simulink model "vertical_smm_3d_with_xz_lqr_with_torque_cmds"  (R2015a)
settings: Solver=FixedStepDiscrete  SolverMode=SingleTasking  StartTime=0.0  StopTime=inf  FixedStep=sample_time  RelTol=1e-3
values from neighbouring files (symbols this model uses):
  forward_dx_of_dxstar = [-1.33147741515 -1.28147741462 -1.23147741409 -1.18147741356 -1.13147741303 -1.0814774125 -1.03147741197 -0.981477411445 -0.931477410916 -0.881477410388 -0.831477409975 -0.781477409737 ... (28413 elements, 41x21x33)]    [ref_trajs.mat]
  forward_x_of_dxstar = [0.245075236011 0.237749717983 0.230424199955 0.223098681927 0.215773163898 0.20844764587 0.201122127842 0.193796609813 0.186471091785 0.179145573757 0.171820055745 0.164494537786 ... (28413 elements, 41x21x33)]    [ref_trajs.mat]
  target_dx_range = [-1 -0.95 -0.9 -0.85 -0.8 -0.75 -0.7 -0.65 -0.6 -0.55 -0.5 -0.45 ... (41 elements, 1x41)]    [ref_trajs.mat]
undefined symbols (not defined in the file or in its folder): A_kalman_fourbar_gear, A_kalman_transverse, A_kalman_vertical, A_lpf_accelerometer, A_lpf_dtau, A_lpf_fourbar_angles, A_lpf_imu, A_lpf_lateral_angle, A_lpf_leg_spring, B1_lpf_accelerometer, B1_lpf_dtau, B1_lpf_fourbar_angles, B1_lpf_imu, B1_lpf_lateral_angle, B1_lpf_leg_spring, B2_lpf_accelerometer, B2_lpf_dtau, B2_lpf_fourbar_angles, B2_lpf_imu, B2_lpf_lateral_angle, B2_lpf_leg_spring, B_dx_versus_x0, B_kalman_fourbar_gear, B_kalman_transverse, B_kalman_vertical, backwards_K_sag_of_t, backwards_P_sag_of_t, C_kalman_fourbar_gear, C_kalman_transverse, C_kalman_vertical, com_leg_motor, com_torso, contact_threshold, control_start_time, d_ankle_to_foot, d_vertical_com, desired_com_forward_velocity, desired_com_lateral_velocity, desired_initial_leg_roll_left, desired_initial_leg_roll_right, desired_stance_beta2, desired_standing_torso_pitch, desired_standing_torso_roll, desired_standing_z, desired_torso_pitch, desired_torso_roll, Discrete, enable_bouncing, enable_hopping, fcut_contact, g, HIP_MTR_MAX_CONT_TORQUE, HIP_MTR_MAX_TORQUE, i_leg_motor, i_robot, i_torso, initial_dx_estimate, initial_dy_estimate, initial_dz_estimate, initial_leg_selection ... (+77)
libraries: simulink x18, ctrlSharedLib x7
(part 5 of 5)

== matlab function vertical_smm_3d_with_xz_lqr_with_torque_cmds/Control/Behavior Control/Primary and Lateral Behavior/Stance/3D Inverse Dynamics yawed ==
  data: right_or_left input; primary_leg_torque output double size=1; torso_roll input double size=2; torso_pitch input double size=2; torso_yaw input size=2; primary_sagittal_leg_angle input size=2; primary_leg_length input size=2; primary_leg_roll input size=2; secondary_leg_roll input size=2; GRF_desired input double size=3; ddRoll_desired input double size=1; g parameter; primary_lateral_torque output double size=1; secondary_lateral_torque output double size=1; primary_leg_force output double size=1; m_leg_motor parameter; m_torso parameter; i_torso parameter; i_leg_motor parameter; lateral_offset parameter; com_torso parameter; torso_centerline_roll_offset_angle parameter
%% Inverse dynamics
function [primary_leg_torque, primary_lateral_torque, secondary_lateral_torque, primary_leg_force]  =  InverseDynamics3D(right_or_left,...
                                                                                                                         torso_roll, torso_pitch, torso_yaw, ...
                                                                                                                         primary_sagittal_leg_angle, primary_leg_length, ...
                                                                                                                         primary_leg_roll, secondary_leg_roll, ...
                                                                                                                         GRF_desired, ddRoll_desired, ...
                                                                                                                         g, m_leg_motor, m_torso, i_torso, i_leg_motor, lateral_offset, com_torso, torso_centerline_roll_offset_angle)

    d = norm(com_torso(2:3));
    It = mean(i_torso);
    Im = mean(i_leg_motor);
    
    phi    = torso_roll(1) + torso_centerline_roll_offset_angle; % roll
    theta  = torso_pitch(1);                   % pitch
    alpha1 = primary_sagittal_leg_angle(1);    % primary sagittal leg angle
    beta1  = primary_leg_roll(1);              % primary leg roll
    beta2  = secondary_leg_roll(1);            % secondary leg roll
    if right_or_left
        beta1 = beta1 - torso_centerline_roll_offset_angle;
        beta2 = beta2 + torso_centerline_roll_offset_angle;
    else
        beta1 = beta1 + torso_centerline_roll_offset_angle;
        beta2 = beta2 - torso_centerline_roll_offset_angle;
    end 
    l1     = primary_leg_length(1);            % primary leg length
    
    dphi    = torso_roll(2);
    dtheta  = torso_pitch(2);
    dpsi    = torso_yaw(2);
    dalpha1 = primary_sagittal_leg_angle(2);
    dbeta1  = primary_leg_roll(2);
    dbeta2  = secondary_leg_roll(2);
    dl1     = primary_leg_length(2);

    Fx = GRF_desired(1);
    Fy = GRF_desired(2);
    Fz = GRF_desired(3);
    ddphi = ddRoll_desired;

    if right_or_left == 1
      A = A_id_roll_yawed_right(lateral_offset,d,m_leg_motor,m_torso,It,Im,phi,theta,alpha1,beta1,beta2,l1);     
      B = B_id_roll_yawed_right(lateral_offset,d,g,m_leg_motor,m_torso,It,Im,phi,theta,alpha1,beta1,beta2,l1,dphi,dtheta,dpsi,dalpha1,dbeta1,dbeta2,dl1,Fx,Fy,Fz,ddphi);
    else
      A = A_id_roll_yawed_left(lateral_offset,d,m_leg_motor,m_torso,It,Im,phi,theta,alpha1,beta1,beta2,l1);     
      B = B_id_roll_yawed_left(lateral_offset,d,g,m_leg_motor,m_torso,It,Im,phi,theta,alpha1,beta1,beta2,l1,dphi,dtheta,dpsi,dalpha1,dbeta1,dbeta2,dl1,Fx,Fy,Fz,ddphi);
    end        
    
    x_id_roll = A \ B;
    primary_leg_torque = x_id_roll(10);
    primary_lateral_torque = x_id_roll(11);
    secondary_lateral_torque = x_id_roll(12);
    primary_leg_force = x_id_roll(13);
end

== matlab function vertical_smm_3d_with_xz_lqr_with_torque_cmds/Control/Behavior Control/Primary and Lateral Behavior/Stance/COM X,Y,Z  trajectory generation ==
  data: stance input; hopping input; bouncing input; x_0 output size=1; y_0 output size=1; z_ref output size=1; dz_ref output size=1; ddz_ref output size=1; x_ref output size=1; dx_ref output size=1; y_ref output size=1; dy_ref output size=1; t input size=1; dx0 input; dy0 input; target_DX input; target_DY input; z_rest_new parameter; z_amplitude parameter; spring_frequency parameter; phase_0 parameter; forward_x_of_dxstar parameter; forward_dx_of_dxstar parameter; target_dx_range parameter; T_s parameter; desired_standing_z parameter; standing_bounce_amplitude parameter; standing_bounce_w input; standing_bounce_dw input
%% COM trajectory generation for stance & foot placement for flight

% Outputs:
% x_0: desired x position for COM at touchdown
% y_0: desired y position for COM at touchdown
% [z_ref, dz_ref, ddz_ref]: reference trajectory for vertical
% [x_ref, dx_ref]: reference trajectory for forward
% [y_ref, dy_ref]: reference trajectory for lateral

% Inputs:
% t: time since touchdown
% dx0: touchdown x velocity
% dy0: touchdown y velocity
% target_DX: desired x velocity at takeoff
% s_duration: nominal stance time
% z_rest_new: z height of oscillation
% target_dx_range: full range of possible x velocities in lookup table
% forward_x_of_dxstar: master lookup table for x trajectories
% T_s: tabled vector from 0 to s_duration

function [x_0, y_0,...
          z_ref, dz_ref, ddz_ref, ...
          x_ref, dx_ref, y_ref, dy_ref] ...
          = ReferenceTrajectory(stance, hopping, bouncing, t, dx0, dy0, target_DX, target_DY, z_rest_new, z_amplitude, ...
            spring_frequency, phase_0, forward_x_of_dxstar, forward_dx_of_dxstar, ...
            target_dx_range, T_s,...
            desired_standing_z, standing_bounce_amplitude, standing_bounce_w, standing_bounce_dw)
    
    % Z trajectory 
    z_ref =  z_rest_new + z_amplitude*sin(spring_frequency*t+phase_0);
    dz_ref = z_amplitude*spring_frequency*cos(spring_frequency*t+phase_0);
    ddz_ref = -z_amplitude*spring_frequency^2*sin(spring_frequency*t+phase_0);
    
    % saturate t and initial velocity to reference library
    t_sat = max( min(t, T_s(end)), 0);

    % [X, dX] trajectory from 0 to s_duration
    forward_x_given_dxstar = squeeze(interp1(target_dx_range, forward_x_of_dxstar, target_DX));
    forward_dx_given_dxstar = squeeze(interp1(target_dx_range, forward_dx_of_dxstar, target_DX));

    dx0 = max( min(dx0, max(forward_dx_given_dxstar(:,1))), min(forward_dx_given_dxstar(:,1)) );
    x_ref  = interp2(T_s, forward_dx_given_dxstar(:,1), forward_x_given_dxstar, t_sat, dx0);
    dx_ref = interp2(T_s, forward_dx_given_dxstar(:,1), forward_dx_given_dxstar, t_sat, dx0);
    x_0 = interp1(forward_dx_given_dxstar(:,1), forward_x_given_dxstar(:,1), dx0);

    % [Y, dY] trajectory from 0 to s_duration
    % Y uses same library as X
    forward_y_given_dxstar = squeeze(interp1(target_dx_range, forward_x_of_dxstar, target_DY));
    forward_dy_given_dxstar = squeeze(interp1(target_dx_range, forward_dx_of_dxstar, target_DY));

    dy0 = max( min(dy0, max(forward_dy_given_dxstar(:,1))), min(forward_dy_given_dxstar(:,1)) );
    y_ref  = interp2(T_s, forward_dy_given_dxstar(:,1), forward_y_given_dxstar, t_sat, dy0);
    dy_ref = interp2(T_s, forward_dy_given_dxstar(:,1), forward_dy_given_dxstar, t_sat, dy0);
    y_0 = interp1(forward_dy_given_dxstar(:,1), forward_y_given_dxstar(:,1), dy0);
    
    if ~hopping && ~bouncing % Standing still
        z_ref = desired_standing_z;
        dz_ref = 0;
        ddz_ref = 0;
        x_ref = 0;
        dx_ref = 0;
        y_ref = 0;
        dy_ref =0;
    elseif ~hopping && bouncing % Bouncing while standing
        z_ref = z_rest_new + standing_bounce_amplitude*sin(t*standing_bounce_w);
        dz_ref = standing_bounce_amplitude*cos(t*standing_bounce_w)*(t*standing_bounce_dw + standing_bounce_w);
        ddz_ref = standing_bounce_amplitude*(2*standing_bounce_dw*cos(t*standing_bounce_w) - (t*standing_bounce_dw + standing_bounce_w)^2*sin(t*standing_bounce_w));
        x_ref = 0;
        dx_ref = 0;
        y_ref = 0;
        dy_ref =0;
    elseif ~stance % Flight
        z_ref = 0;
        dz_ref = 0;
        ddz_ref = 0;
        x_ref = 0;
        dx_ref = 0;
        y_ref = 0;
        dy_ref =0;    
    end
  
end

== matlab function vertical_smm_3d_with_xz_lqr_with_torque_cmds/Control/Behavior Control/Primary and Lateral Behavior/Stance/Feedback for Lateral Stabilization ==
  data: feedforward_Fy output; hopping input; stance input; right_left input; rolldroll input; primary_lateral_torque_desired output; symdsym input; beta1dbeta1 input; beta2dbeta2 input; ydy_ref input; zdzddz_ref input; GRF_measured input; secondary_lateral_torque_desired output double size=1; m_torso parameter; m_leg_motor parameter; m_leg parameter; lateral_offset parameter; com_torso parameter; i_torso parameter; i_leg_motor parameter; desired_standing_torso_roll parameter; desired_torso_roll parameter; desired_stance_beta2 parameter; angular_momentum output; k_stance_torso_roll parameter; k_stance_secondary_roll parameter; g parameter; m_total_real parameter
%  x_front = [y, roll, sym, dy, droll, L]; 
function [feedforward_Fy, primary_lateral_torque_desired, secondary_lateral_torque_desired, angular_momentum]  =  ...
    FrontalStabilization(hopping, stance, right_left, rolldroll, symdsym, beta1dbeta1, beta2dbeta2, ydy_ref, zdzddz_ref, GRF_measured,...
           m_torso, m_leg_motor, m_leg, lateral_offset, com_torso, i_torso, i_leg_motor, ...
           desired_standing_torso_roll, desired_torso_roll, desired_stance_beta2, k_stance_torso_roll, k_stance_secondary_roll, g, m_total_real)
    
    % Angular momentum about the pelvis in the frontal plane
    d = norm(com_torso(2:3));
    It_f = i_torso(1);
    Im_f = i_leg_motor(1);
    angular_momentum = rolldroll(2)*(m_torso*d^2 + It_f + 2*(m_leg_motor*lateral_offset^2+ Im_f)) -symdsym(2)*(m_leg_motor*lateral_offset^2+Im_f);
    
    % Feedforward GRFy for inverse dynamics
    Fz_ref = (zdzddz_ref(3)+g)*m_total_real;
    feedforward_Fy = Fz_ref*ydy_ref(1)/zdzddz_ref(1);
    feedforward_Fy = min(max(feedforward_Fy, -0.5*abs(GRF_measured(3))), 0.5*abs(GRF_measured(3)));
    
    % Desired states
    if hopping
        desired_torso_roll_state = [desired_torso_roll; 0]; 
    else
        desired_torso_roll_state = [desired_standing_torso_roll; 0];
    end
    desired_beta2_state = [desired_stance_beta2; 0];
    
    % Motor torque commands
    ddz = GRF_measured(3) / m_total_real - g;
    gravity_comp = (m_leg_motor+m_leg)*lateral_offset*ddz;
    contact_factor = max(min(GRF_measured(3)/(m_total_real*g),1.0),0);
    secondary_lateral_torque_desired = k_stance_secondary_roll*(desired_beta2_state - beta2dbeta2);
    primary_lateral_feedback = contact_factor*k_stance_torso_roll*(desired_torso_roll_state - rolldroll);
    if right_left % Right leg beta direction is opposite torso roll
        primary_lateral_feedback = -primary_lateral_feedback;
    end
    primary_lateral_torque_desired =  primary_lateral_feedback + secondary_lateral_torque_desired;
      
    if ~stance
        primary_lateral_torque_desired = 0;
        secondary_lateral_torque_desired = 0;
        feedforward_Fy = 0;
    end
end

== matlab function vertical_smm_3d_with_xz_lqr_with_torque_cmds/Control/Behavior Control/Primary and Lateral Behavior/Stance/LQR Feedback for Desired Forward GRF ==
  data: hopping input; stance input; GRFx_desired output; netural_pitch_ff output; true_ff output; GRFx_lqr output; ddtheta_star output; ddtheta_star_neutral output; xdx input; thetadtheta input; zdz input; Fz input; xdx_ref input size=2; theta_star input; K_sag input; P_sag input; measured_GRF input; Fx_disturbance input; i_robot parameter; cost_to_go output double size=1; ang_mom output; desired_standing_torso_pitch parameter; k_LQR_sagittal_infinite parameter; P_LQR_sagittal_infinite parameter
%% LQR for x state

% stance: 1 if in stance, 0 otherwise
% xdx: [ x from stance leg to COM, dx of COM]
% thetadtheta: [pitch, dpitch]
% zdz: [z of COM, dz of COM]
% Fz: Desired z GRF
% xdx_ref: [x, dx] current reference point for COM
% theta_star: desired torso pitch
% K_sag: time dependent LQR gain


% sagittal_state: [x, pitch, dx, dptich]
% theta_star: desired torso pitch


function [GRFx_desired, netural_pitch_ff, true_ff, GRFx_lqr, ddtheta_star, ddtheta_star_neutral, cost_to_go, ang_mom]  =  ...
    LQR_Sagittal(hopping, stance, xdx, thetadtheta, zdz, Fz, xdx_ref, theta_star, K_sag, P_sag, measured_GRF, Fx_disturbance, i_robot,...
    desired_standing_torso_pitch, k_LQR_sagittal_infinite, P_LQR_sagittal_infinite)


    sagittal_state = [xdx(1); thetadtheta(1); xdx(2); thetadtheta(2)];
    netural_pitch_ff = Fz*xdx(1)/zdz(1);
    true_ff = Fz*xdx_ref(1)/zdz(1);
    
    if hopping
        sagittal_reference = [xdx_ref(1), theta_star, xdx_ref(2), 0]';
        sagittal_error = (sagittal_state - sagittal_reference);
        cost_to_go = 0.5*sagittal_error'*P_sag*sagittal_error;
        GRFx_lqr = - K_sag*sagittal_error;
        GRFx_desired = true_ff + GRFx_lqr;
    else
        sagittal_reference = [xdx_ref(1), desired_standing_torso_pitch, xdx_ref(2), 0]';
        sagittal_error = (sagittal_state - sagittal_reference);
        cost_to_go = 0.5*sagittal_error'*P_LQR_sagittal_infinite*sagittal_error;
        %GRFx_desired = i_robot/zdz(1)*(150*(thetadtheta(1)-desired_standing_torso_pitch) + 30*thetadtheta(2)) + netural_pitch_ff;
        GRFx_lqr = - k_LQR_sagittal_infinite*sagittal_error;
        GRFx_desired = GRFx_lqr;
    end
    
    GRFx_desired = GRFx_desired - Fx_disturbance;
    GRFx_desired = min(max(GRFx_desired, -0.5*abs(measured_GRF(3))), 0.5*abs(measured_GRF(3))); % saturate to friction cone
    
    if stance == 0
      GRFx_lqr = 0;
      cost_to_go = 0;
      netural_pitch_ff = 0;
      true_ff = 0;
    end
    
    % quantities for logging
    ddtheta_star_neutral = -(GRFx_lqr)*zdz(1)/i_robot;
    ddtheta_star = -(GRFx_desired - netural_pitch_ff)*zdz(1)/i_robot;
    ang_mom = i_robot*thetadtheta(2);
end

== matlab function vertical_smm_3d_with_xz_lqr_with_torque_cmds/Control/Behavior Control/Primary and Lateral Behavior/Stance/LQR Feedback for Desired Vertical GRF ==
  data: hopping input; stance input; zdzddz_ref input size=3; GRFz_desired output; GRFz_feedforward output; z_state input; leg_length input; Fz_disturbance input; k_LQR_vertical parameter; P_LQR_vertical parameter; k_vertical_winch parameter; m_total_real parameter; g parameter; cost_to_go output double size=1; max_leg_length parameter
%% LQR for z during stance

% stance: 1 if in stance, 0 otherwise
% z_state: [z, dz] current estimate
% zdzddz_ref: reference trajectory for z position, velocity, and acceleration


% GRFz_desired: desired z GRF
% cost_to_go: remaining LQR cost

function [GRFz_desired, GRFz_feedforward, cost_to_go]   =  ...
               LQR_Vertical_Height(hopping, stance, zdzddz_ref, z_state, leg_length, Fz_disturbance,...
                                   k_LQR_vertical, P_LQR_vertical, k_vertical_winch, m_total_real, g, max_leg_length)

    z_ref = zdzddz_ref(1:2);     
    ddz_ref = zdzddz_ref(3);
    z_error = (z_state - z_ref);
    GRFz_feedforward = m_total_real*(g+ddz_ref);
    GRFz_desired = GRFz_feedforward - k_LQR_vertical*z_error;
    GRFz_desired = GRFz_desired - Fz_disturbance;
    
    if hopping
        if z_ref(2) < 0
            GRFz_desired = max(50, GRFz_desired); % prevent foot from slipping
        elseif leg_length(1) >= max_leg_length
            GRFz_desired = 0; % prevent hyperextension
        end
    else
        GRFz_desired = GRFz_feedforward - k_vertical_winch*z_error;
        GRFz_desired = GRFz_desired - Fz_disturbance;
        GRFz_desired = max(200, GRFz_desired);
    end
    
    cost_to_go = z_error'*P_LQR_vertical*z_error;
    
    if stance == 0
      GRFz_desired = 0;
      cost_to_go = 0;
    end
end

== matlab function vertical_smm_3d_with_xz_lqr_with_torque_cmds/Control/Behavior Control/Primary and Lateral Behavior/Stance/Lookup finite horizon LQR gain ==
  data: K_sag output size=[1,4]; P_sag output size=[4,4]; t_forward input; backwards_K_sag_of_t parameter; T_lqr parameter; stance_duration parameter; backwards_P_sag_of_t parameter
%% Interpolates pregenerated finite horizon LQR gain tables 
% sagittal_state: [X, Pitch, dX, dPtich]
% frontal state: [Y; Roll; sym; dY; dRoll; angular_momentum];
function [K_sag, P_sag]  =  FiniteHorizonLQRLookup(t_forward, backwards_K_sag_of_t, T_lqr, stance_duration, backwards_P_sag_of_t)
  t = stance_duration - t_forward; % gains are scheduled w.r.t time until end.                                     
  t = min(max(t, min(T_lqr)), max(T_lqr));
  K_sag = interp1(T_lqr, backwards_K_sag_of_t, t);
  P_sag = squeeze(interp1(T_lqr,backwards_P_sag_of_t,t));
end

== matlab function vertical_smm_3d_with_xz_lqr_with_torque_cmds/Control/Behavior Control/Primary and Lateral Behavior/Stance/X & Pitch State Disturbance Observer ==
  data: enabled input; Fx input size=1; z_dz input; d_hat_tp1 output size=1; x_dx input size=2; theta_dtheta input; sample_time parameter; m_total_real parameter; g parameter; i_robot parameter
function d_hat_tp1 = disturbance_observer(enabled, Fx, z_dz, x_dx, theta_dtheta, sample_time, m_total_real, g, i_robot)
    
    order = 1;
    L = 2*2.^[1:order+1] .* factorial(order+1)./(factorial(order+1-(1:(order+1))).*factorial(1:order+1));

    persistent z_t d_hat_t integral_term;
    if isempty(z_t) || enabled
        z_t = 0;
        d_hat_t = 0;
        integral_term = zeros(order,1);
    end
    
%     persistent z_t;
%     if isempty(z_t) || enabled
%         z_t = 0;
%     end

    % Define system
    A_d = [ 1, 0, sample_time, 0;
            0, 1, 0, sample_time;
            0, 0, 1, 0;
            m_total_real*g*sample_time/i_robot, 0, 0, 1];
    Bu_d = [0; 0; sample_time/m_total_real; -sample_time*z_dz(1)/i_robot];
    A_c = [ 0, 0, 1, 0;
            0, 0, 0, 1;
            0, 0, 0, 0;
            m_total_real*g/i_robot, 0, 0, 0];
    Bu_c = [0; 0; 1/m_total_real; -z_dz(1)/i_robot];
    Bd_c = [0; 0; 1/m_total_real; -z_dz(1)/i_robot];
    %L = L_dob_xdx_thetadtheta;
    x = [x_dx(1); theta_dtheta(1); x_dx(2); theta_dtheta(2)];
    u = Fx;

%     % Estimate disturbance
%     x_tp1 = A_d*x + Bu_d*u;
%     z_tp1 = z_t - sample_time*L*(Bd_c*(z_t + L*x) + A_c*x + Bu_c*u);
%     d_hat_tp1 = z_tp1 + L*x_tp1;
%     z_t = z_tp1;

    % Estimate disturbance
    z_tp1 = z_t + sample_time*(pinv(Bd_c)*(A_c*x + Bu_c*u) + d_hat_t);
    x_tp1 = A_d*x + Bu_d*u;
    integral_term(1) = integral_term(1) + sample_time*(pinv(Bd_c)*x_tp1 - z_tp1);
    for i=2:order
        integral_term(i) = integral_term(i) + sample_time*integral_term(i-1);
    end
    d_hat_tp1 = L*[(pinv(Bd_c)*x_tp1 - z_tp1); integral_term];
    d_hat_t = d_hat_tp1;
    z_t = z_tp1;
    
    
end

== matlab function vertical_smm_3d_with_xz_lqr_with_torque_cmds/Control/Behavior Control/Primary and Lateral Behavior/Stance/Z State Disturbance Observer Error-Proportional - 1st order ==
  data: enabled input; Fz input size=1; d_hat_tp1 output size=1; z_dz input size=2; m_total_real parameter; g parameter; sample_time parameter
function d_hat_tp1  = disturbance_observer(enabled, Fz, z_dz, m_total_real, g, sample_time)

    order = 1;
    L = 2*2.^[1:order+1] .* factorial(order+1)./(factorial(order+1-(1:(order+1))).*factorial(1:order+1));

    persistent z_t d_hat_t integral_term;
    if isempty(z_t) || enabled
        z_t = 0;
        d_hat_t = 0;
        integral_term = zeros(order,1);
    end
   
    % Define system
    A_d = [1, sample_time; 0, 1];
    Bu_d = [0; sample_time/m_total_real];
    A_c = [0 1; 0 0];
    Bu_c = [0; 1/m_total_real];
    Bd_c = [0; 1/m_total_real];
    x = z_dz;
    u = Fz - m_total_real*g;
 
    % Estimate disturbance
    z_tp1 = z_t + sample_time*(pinv(Bd_c)*(A_c*x + Bu_c*u) + d_hat_t);
    x_tp1 = A_d*x + Bu_d*u;
    integral_term(1) = integral_term(1) + sample_time*(pinv(Bd_c)*x_tp1 - z_tp1);
    for i=2:order
        integral_term(i) = integral_term(i) + sample_time*integral_term(i-1);
    end
    d_hat_tp1 = L*[(pinv(Bd_c)*x_tp1 - z_tp1); integral_term];
    d_hat_t = d_hat_tp1;
    z_t = z_tp1;
    
end

== matlab function vertical_smm_3d_with_xz_lqr_with_torque_cmds/Control/Behavior Control/Primary and Lateral Behavior/Stance/Z State Disturbance Observer Error-Proportional - 2nd order ==
  data: enabled input; Fz input size=1; d_hat_tp1 output size=1; z_dz input size=2; m_total_real parameter; g parameter; sample_time parameter
function d_hat_tp1  = disturbance_observer(enabled, Fz, z_dz, m_total_real, g, sample_time)

    order = 2;
    L = 2*2.^[1:order+1] .* factorial(order+1)./(factorial(order+1-(1:(order+1))).*factorial(1:order+1));

    persistent z_t d_hat_t integral_term;
    if isempty(z_t) || enabled
        z_t = 0;
        d_hat_t = 0;
        integral_term = zeros(order,1);
    end
   
    % Define system
    A_d = [1, sample_time; 0, 1];
    Bu_d = [0; sample_time/m_total_real];
    A_c = [0 1; 0 0];
    Bu_c = [0; 1/m_total_real];
    Bd_c = [0; 1/m_total_real];
    x = z_dz;
    u = Fz - m_total_real*g;
 
    % Estimate disturbance
    z_tp1 = z_t + sample_time*(pinv(Bd_c)*(A_c*x + Bu_c*u) + d_hat_t);
    x_tp1 = A_d*x + Bu_d*u;
    integral_term(1) = integral_term(1) + sample_time*(pinv(Bd_c)*x_tp1 - z_tp1);
    for i=2:order
        integral_term(i) = integral_term(i) + sample_time*integral_term(i-1);
    end
    d_hat_tp1 = L*[(pinv(Bd_c)*x_tp1 - z_tp1); integral_term];
    d_hat_t = d_hat_tp1;
    z_t = z_tp1;
    
end

== matlab function vertical_smm_3d_with_xz_lqr_with_torque_cmds/Control/Behavior Control/Primary and Lateral Behavior/ToggleRightLeftLeg ==
  data: toggle input boolean; direction output double; previous input double
function direction = TogglePositiveNegative(toggle, previous)
    
    if toggle
        direction = -previous;
    else
        direction = previous;
    end

end

== matlab function vertical_smm_3d_with_xz_lqr_with_torque_cmds/Control/Compute Body Frame Accelerations/Convert to Body Frame IMU Accelerations ==
  data: accelerometer input; imu_accelerations output; g parameter
function imu_accelerations = imu_to_body_frame(accelerometer, g)
    z_up_rotation = [1, 0, 0; 0, 0, 1; 0, -1, 0];
    align_xy_rotation = [sqrt(2)/2, -sqrt(2)/2, 0; sqrt(2)/2, sqrt(2)/2, 0; 0, 0, 1];
    imu_accelerations = g*z_up_rotation*align_xy_rotation*accelerometer;
end

== matlab function vertical_smm_3d_with_xz_lqr_with_torque_cmds/Control/Behavior Control/Compute COM Translational Acceleration ==
  data: angular_velocities input; com_acceleration_yawed output; angular_accelerations input; translational_accelerations input; torso_roll input; torso_pitch input; pelvis_to_com input; pelvis_to_imu parameter; g parameter
function com_acceleration_yawed = compute_com_acceleration(angular_velocities, angular_accelerations, translational_accelerations, torso_roll, torso_pitch, pelvis_to_com, pelvis_to_imu, g)

    imu_to_com = pelvis_to_com - pelvis_to_imu';
    com_acceleration_body = translational_accelerations + cross(angular_accelerations, imu_to_com) + cross(angular_velocities, cross(angular_velocities, imu_to_com));
    com_acceleration_yawed = R_pitch(torso_pitch(1))*R_roll(torso_roll(1))*com_acceleration_body;
    com_acceleration_yawed(3) = com_acceleration_yawed(3) - g;
end
function R_pr = R_roll(phi) % map from rolled to pitched
  R_pr = [1 0 0; 0 cos(phi) -sin(phi); 0 sin(phi) cos(phi)]; 
end
function R_yp = R_pitch(theta) % map from pitched to yawed
  R_yp = [cos(theta), 0, sin(theta); 0 1 0; -sin(theta), 0, cos(theta)];
end

== matlab function vertical_smm_3d_with_xz_lqr_with_torque_cmds/Control/Behavior Control/State Estimation/Kalman Filtering/Measurement Noise Covariance Matricies ==
  data: R_transverse output; vertical_GRF_L input; vertical_GRF_R input; R_kalman_foot_stance parameter; R_kalman_foot_slip parameter; R_kalman_accelerometer parameter; sample_time parameter; m_total_real parameter; g parameter; R_vertical output; kalman_stance_slip_threshold parameter
function [R_transverse, R_vertical] =...
         MeasurementNoiseCovariance(vertical_GRF_L, vertical_GRF_R, ...
           R_kalman_foot_stance, R_kalman_foot_slip, R_kalman_accelerometer, sample_time, m_total_real, g, kalman_stance_slip_threshold)

    % filter states: [dx_w]; [dy_w]; [dz_w];
    % measurements:  [dx_w-dfL + dfL_hat; dx_w-dfR + dfR_hat]; 

    ratio_L = max(0, min(vertical_GRF_L/(kalman_stance_slip_threshold*m_total_real*g),1)); % ratio is 0 if no load, 1 if at least equilibrium
    ratio_R = max(0, min(vertical_GRF_R/(kalman_stance_slip_threshold*m_total_real*g),1));
    R_transverse = diag([ratio_L*R_kalman_foot_stance + (1-ratio_L)*R_kalman_foot_slip, ...
                         ratio_R*R_kalman_foot_stance + (1-ratio_R)*R_kalman_foot_slip, ...
                         R_kalman_accelerometer])/sample_time;
    R_vertical = diag([ratio_L*R_kalman_foot_stance  + (1-ratio_L)*R_kalman_foot_slip,...
                       ratio_R*R_kalman_foot_stance  + (1-ratio_R)*R_kalman_foot_slip,...
                       R_kalman_accelerometer])/sample_time;
end

== matlab function vertical_smm_3d_with_xz_lqr_with_torque_cmds/Control/Behavior Control/State Estimation/Kalman Filtering/eigen values ==
  data: Z input; E output
function E = eigen(Z)
    E = real(eig(Z));
    E = sort(E);
end

== matlab function vertical_smm_3d_with_xz_lqr_with_torque_cmds/Control/Behavior Control/State Estimation/Kalman Filtering/eigen values1 ==
  data: Z input; E output
function E = eigen(Z)
    E = real(eig(Z));
    E = sort(E);
end

== matlab function vertical_smm_3d_with_xz_lqr_with_torque_cmds/Control/Behavior Control/State Estimation/Kalman Filtering/eigen values2 ==
  data: Z input; E output
function E = eigen(Z)
    E = real(eig(Z));
    E = sort(E);
end

== matlab function vertical_smm_3d_with_xz_lqr_with_torque_cmds/Control/Behavior Control/State Estimation/PositionUsingRobotGeometry ==
  data: com_left_foot output; dcom_left_foot output; com_right_foot output; dcom_right_foot output; right_left input; horizontal_com_position output; roll input; pitch input; yaw input; horizontal_com_velocity output; lateral_com_position output; lateral_com_velocity output; left_leg_sagittal_angle input; left_leg_lateral_angle input; left_leg_length input; right_leg_sagittal_angle input; right_leg_lateral_angle input; right_leg_length input; m_torso parameter; m_leg_motor parameter; m_leg parameter; com_torso parameter; com_leg_motor parameter; lateral_offset parameter; vertical_com_position output; vertical_com_velocity output; com_pelvis output; dcom_pelvis output
% Returns 2D COM relative to primary foot
function [com_left_foot, dcom_left_foot, com_right_foot, dcom_right_foot,...
          horizontal_com_position, horizontal_com_velocity, ...
          lateral_com_position, lateral_com_velocity, ...
          vertical_com_position, vertical_com_velocity, ...
          com_pelvis, dcom_pelvis] = ...
         ComPositionUsingRobotGeometry(right_left, ...
                                    roll, pitch, yaw, ...
                                    left_leg_sagittal_angle, left_leg_lateral_angle, left_leg_length, ...
                                    right_leg_sagittal_angle, right_leg_lateral_angle, right_leg_length, ...
                                    m_torso, m_leg_motor, m_leg, com_torso, com_leg_motor, lateral_offset)
                    
    q =  [roll(1), pitch(1), yaw(1), left_leg_sagittal_angle(1), left_leg_lateral_angle(1), left_leg_length(1), right_leg_sagittal_angle(1), right_leg_lateral_angle(1), right_leg_length(1)];
    dq = [roll(2), pitch(2), yaw(2), left_leg_sagittal_angle(2), left_leg_lateral_angle(2), left_leg_length(2), right_leg_sagittal_angle(2), right_leg_lateral_angle(2), right_leg_length(2)];
                    
    [ com_pelvis, dcom_pelvis, ...
      com_left_foot, dcom_left_foot, ...
      com_right_foot, dcom_right_foot ] = ...
    ComCalculationFromRobot( q, dq, m_torso, m_leg_motor, m_leg, com_torso, com_leg_motor, lateral_offset );

    if right_left
        com_position = com_right_foot(4:6);
        com_velocity = dcom_right_foot(4:6);
    else
        com_position = com_left_foot(4:6);
        com_velocity = dcom_left_foot(4:6);
    end


    horizontal_com_position = com_position(1);
    horizontal_com_velocity = com_velocity(1);
    lateral_com_position = com_position(2);
    lateral_com_velocity = com_velocity(2);
    vertical_com_position = com_position(3);
    vertical_com_velocity = com_velocity(3);

end
